simulink model "FlOWCITSS_3dof"  (R2019a)
settings: Solver=FixedStepAuto  StartTime=0.0  StopTime=15  FixedStep=0.00001  MaxStep=0.0001  RelTol=1e-5
values from neighbouring files (symbols this model uses):
  a11Inf = addedMassInf(1,4)    [FlOWCITSS.m]
  a13Inf = addedMassInf(2,4)    [FlOWCITSS.m]
  a15Inf = addedMassInf(3,4)    [FlOWCITSS.m]
  a31Inf = addedMassInf(4,4)    [FlOWCITSS.m]
  a33Inf = addedMassInf(5,4)    [FlOWCITSS.m]
  a35Inf = addedMassInf(6,4)    [FlOWCITSS.m]
  a51Inf = addedMassInf(7,4)    [FlOWCITSS.m]
  a53Inf = addedMassInf(8,4)    [FlOWCITSS.m]
  a55Inf = addedMassInf(9,4)    [FlOWCITSS.m]
  AH1 = full(SER.A)    [FlOWCITSS.m]
  AH3 = full(SER.A)    [FlOWCITSS.m]
  AH5 = full(SER.A)    [FlOWCITSS.m]
  AK11 = full(SER.A)    [FlOWCITSS.m]
  AK13 = full(SER.A)    [FlOWCITSS.m]
  AK15 = full(SER.A)    [FlOWCITSS.m]
  AK31 = full(SER.A)    [FlOWCITSS.m]
  AK33 = full(SER.A)    [FlOWCITSS.m]
  AK35 = full(SER.A)    [FlOWCITSS.m]
  AK51 = full(SER.A)    [FlOWCITSS.m]
  AK53 = full(SER.A)    [FlOWCITSS.m]
  AK55 = full(SER.A)    [FlOWCITSS.m]
  AY = full(SER.A)    [FlOWCITSS.m]
  BH1 = SER.B    [FlOWCITSS.m]
  BH3 = SER.B    [FlOWCITSS.m]
  BH5 = SER.B    [FlOWCITSS.m]
  BK11 = SER.B    [FlOWCITSS.m]
  BK13 = SER.B    [FlOWCITSS.m]
  BK15 = SER.B    [FlOWCITSS.m]
  BK31 = SER.B    [FlOWCITSS.m]
  BK33 = SER.B    [FlOWCITSS.m]
  BK35 = SER.B    [FlOWCITSS.m]
  BK51 = SER.B    [FlOWCITSS.m]
  BK53 = SER.B    [FlOWCITSS.m]
  BK55 = SER.B    [FlOWCITSS.m]
  BY = SER.B    [FlOWCITSS.m]
  C1inf = cInf(1,2)    [FlOWCITSS.m]
  C3inf = cInf(1,3)    [FlOWCITSS.m]
  C5inf = cInf(1,4)    [FlOWCITSS.m]
  CH1 = SER.C    [FlOWCITSS.m]
  CH3 = SER.C    [FlOWCITSS.m]
  CH5 = SER.C    [FlOWCITSS.m]
  CK11 = SER.C    [FlOWCITSS.m]
  CK13 = SER.C    [FlOWCITSS.m]
  CK15 = SER.C    [FlOWCITSS.m]
  CK31 = SER.C    [FlOWCITSS.m]
  CK33 = SER.C    [FlOWCITSS.m]
  CK35 = SER.C    [FlOWCITSS.m]
  CK51 = SER.C    [FlOWCITSS.m]
  CK53 = SER.C    [FlOWCITSS.m]
  CK55 = SER.C    [FlOWCITSS.m]
  CY = SER.C    [FlOWCITSS.m]
  DH1 = SER.D    [FlOWCITSS.m]
  DH3 = SER.D    [FlOWCITSS.m]
  DH5 = SER.D    [FlOWCITSS.m]
  DK11 = SER.D    [FlOWCITSS.m]
  DK13 = SER.D    [FlOWCITSS.m]
  DK15 = SER.D    [FlOWCITSS.m]
  DK31 = SER.D    [FlOWCITSS.m]
  DK33 = SER.D    [FlOWCITSS.m]
  DK35 = SER.D    [FlOWCITSS.m]
  DK51 = SER.D    [FlOWCITSS.m]
  DK53 = SER.D    [FlOWCITSS.m]
  DK55 = SER.D    [FlOWCITSS.m]
  DY = SER.D    [FlOWCITSS.m]
  gamma = 1.4    [FlOWCITSS_inputs.m]
  I5 = 1/(4.1625*10^8)    (= 2.4024024024e-09)    [FlOWCITSS_inputs.m]
  Mm = 1/(2.0270*10^6)    (= 4.93339911199e-07)    [FlOWCITSS_inputs.m]
  p0 = 101325    [FlOWCITSS_inputs.m]
  r1 = internalArea*0    (= 0)    [FlOWCITSS_inputs.m]
  r3 = internalArea*1    (= 472.5)    [FlOWCITSS_inputs.m]
  r5 = -internalArea*(5)    (= -2362.5)    [FlOWCITSS_inputs.m]
  Re = 10    [FlOWCITSS_inputs.m]
  Red1 = 91000    [FlOWCITSS_inputs.m]
  Red3 = 619000    [FlOWCITSS_inputs.m]
  Red5 = 190000000    [FlOWCITSS_inputs.m]
  Rq1 = rho*A1*Cd1    (= 1181250)    [FlOWCITSS_inputs.m]
  Rq3 = rho*A3*Cd3    (= 4725000)    [FlOWCITSS_inputs.m]
  Rq5 = 0    [FlOWCITSS_inputs.m]
  Ru = 20    [FlOWCITSS_inputs.m]
  SbS1 = +488000    (= 488000)    [FlOWCITSS_inputs.m]
  SbS3 = hydrostatics.data(15,3)*(rho*g*(ULEN^2))+11100    [FlOWCITSS_inputs.m]
  SbS35 = hydrostatics.data(17,3)*(rho*g*(ULEN^3))    [FlOWCITSS_inputs.m]
  SbS5 = hydrostatics.data(29,3)*(rho*g*(ULEN^4))+9920000    [FlOWCITSS_inputs.m]
  SbS53 = hydrostatics.data(27,3)*(rho*g*(ULEN^3))    [FlOWCITSS_inputs.m]
  V0 = 27*17.5*10    (= 4725)    [FlOWCITSS_inputs.m]
libraries: simulink x13
settings Model: Creator=huffl  LastModifiedBy=huffl
settings SolverCC: ZeroCrossAlgorithm=Adaptive

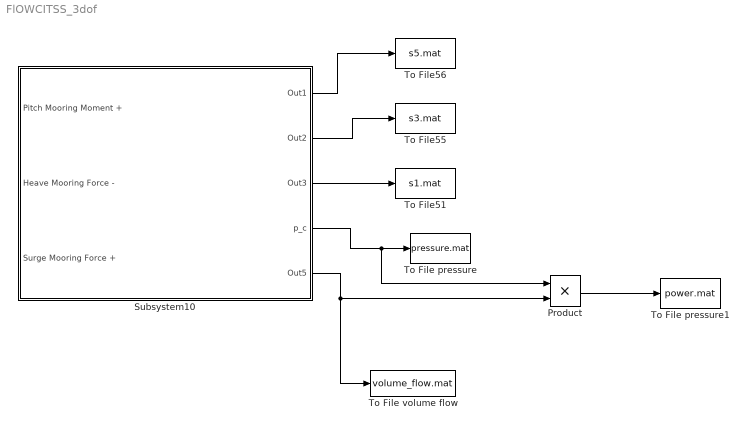
== system FlOWCITSS_3dof ==
  Product : Product
  Subsystem10 : Subsystem
  To File pressure : ToFile  Filename=pressure.mat  MatrixName=p_c  SaveFormat=Timeseries
  To File pressure1 : ToFile  Filename=power.mat  MatrixName=pneumaticPower  SaveFormat=Timeseries
  To File volume flow : ToFile  Filename=volume_flow.mat  MatrixName=Q_turbine  SaveFormat=Timeseries
  To File51 : ToFile  Filename=s1.mat  MatrixName=s1  SaveFormat=Timeseries
  To File55 : ToFile  Filename=s3.mat  MatrixName=s3  SaveFormat=Timeseries
  To File56 : ToFile  Filename=s5.mat  MatrixName=s5  SaveFormat=Timeseries
  wires:
  Subsystem10/1(Out1) -> To File56/1
  Subsystem10/2(Out2) -> To File55/1
  Subsystem10/3(Out3) -> To File51/1
  Subsystem10/4(p_c) -> Product/1, To File pressure/1
  Subsystem10/5(Out5) -> To File volume flow/1, Product/2
  Product/1 -> To File pressure1/1

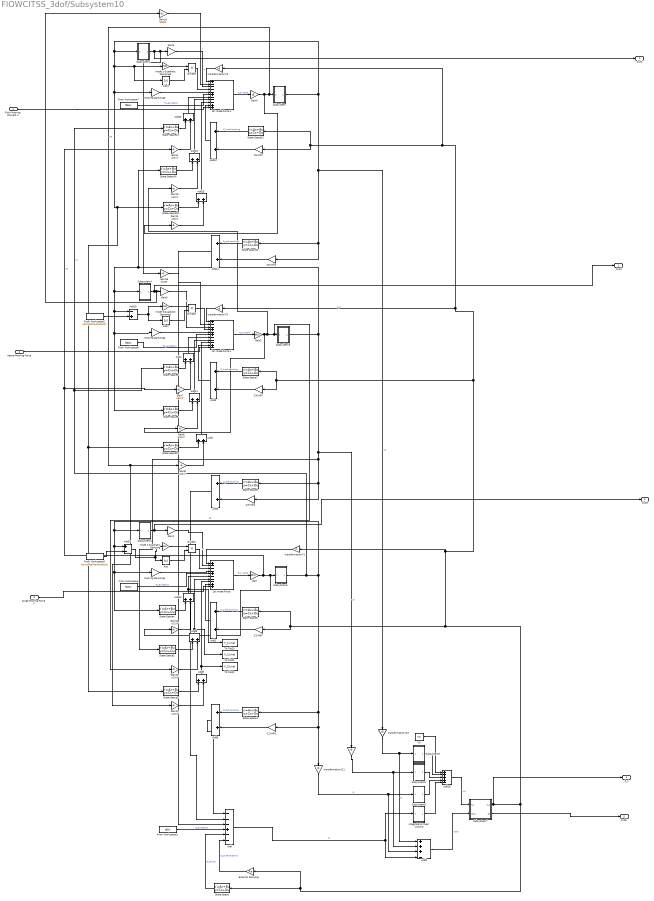
== system FlOWCITSS_3dof/Subsystem10 ==
  Pitch Mooring Moment + : Inport
  Heave Mooring Force - : Inport  Port=2
  "Surge Mooring Force + " : Inport  Port=3
  " " : Gain  Gain=r3
  "1st mode Force " : Sum  Inputs=+---+---++
  1st mode Force 1 : Sum  Inputs=+--+-+---+-
  1st mode Force 2 : Sum  Inputs=+----+---++
  Abs : Abs
  Abs2 : Abs
  Abs3 : Abs
  Add : Sum  Inputs=---+--
  Add{1,3..16} (15 alike) : Sum
  Add18 : Sum  Inputs=++++-
  Add19 : Sum  Inputs=-+
  Add2 : Sum  Inputs=+++-
  Add20 : Sum  Inputs=+-
  C1(inf)F : Gain  Gain=C1inf
  C1(inf)Q : Gain  Gain=C1inf
  C3(inf)F : Gain  Gain=C3inf
  C3(inf)Q : Gain  Gain=C3inf
  C5(inf)F : Gain  Gain=C5inf
  C5(inf)Q : Gain  Gain=C5inf
  Divide1 : Product  Inputs=**
  Divide2 : Product  Inputs=**
  Divide3 : Product  Inputs=**
  External Damping : Gain  Gain=Re
  From Workspace : FromWorkspace  VariableName=f1Exc  SampleTime=0
  From Workspace1 : FromWorkspace  VariableName=qExc  SampleTime=0
  From Workspace2 : FromWorkspace  VariableName=verticalWaveVelocity  SampleTime=0
  From Workspace3 : FromWorkspace  VariableName=horizontalWaveVelocity  SampleTime=0
  From Workspace6 : FromWorkspace  VariableName=f3Exc  SampleTime=0
  From Workspace7 : FromWorkspace  VariableName=f5Exc  SampleTime=0
  Gain : Gain  Gain=Mm
  Gain1 : Gain  Gain=SbS1
  Gain10 : Gain  Gain=a53Inf
  Gain11 : Gain  Gain=a55Inf
  Gain12 : Gain  Gain=a15Inf
  Gain13 : Gain  Gain=a13Inf
  Gain14 : Gain  Gain=a11Inf
  Gain15 : Gain  Gain=SbS35
  Gain16 : Gain  Gain=SbS53
  Gain2 : Gain  Gain=Mm
  Gain3 : Gain  Gain=SbS3
  Gain4 : Gain  Gain=I5
  Gain5 : Gain  Gain=SbS5
  Gain6 : Gain  Gain=a33Inf
  Gain7 : Gain  Gain=a31Inf
  Gain8 : Gain  Gain=a35Inf
  Gain9 : Gain  Gain=a51Inf
  "Integrate to creat Volume " : Subsystem
  Mooring Damping1 : Gain  Gain=Red1
  Mooring Damping2 : Gain  Gain=Red3
  Mooring Damping3 : Gain  Gain=Red5
  State-Space : StateSpace  A=AY  B=BY  C=CY  D=DY  InitialCondition=0
  State-Space1 : StateSpace  A=AH1  B=BH1  C=CH1  D=DH1  InitialCondition=0
  State-Space10 : StateSpace  A=AK35  B=BK35  C=CK35  D=DK35  InitialCondition=0
  State-Space11 : StateSpace  A=AH5  B=BH5  C=CH5  D=DH5  InitialCondition=0
  State-Space12 : StateSpace  A=AH5  B=BH5  C=CH5  D=DH5  InitialCondition=0
  State-Space13 : StateSpace  A=AK51  B=BK51  C=CK51  D=DK51  InitialCondition=0
  State-Space14 : StateSpace  A=AK53  B=BK53  C=CK53  D=DK53  InitialCondition=0
  State-Space15 : StateSpace  A=AK55  B=BK55  C=CK55  D=DK55  InitialCondition=0
  State-Space2 : StateSpace  A=AK15  B=BK15  C=CK15  D=DK15  InitialCondition=0
  State-Space3 : StateSpace  A=AK13  B=BK13  C=CK13  D=DK13  InitialCondition=0
  State-Space4 : StateSpace  A=AK11  B=BK11  C=CK11  D=DK11  InitialCondition=0
  State-Space5 : StateSpace  A=AH1  B=BH1  C=CH1  D=DH1  InitialCondition=0
  State-Space6 : StateSpace  A=AH3  B=BH3  C=CH3  D=DH3  InitialCondition=0
  State-Space7 : StateSpace  A=AH3  B=BH3  C=CH3  D=DH3  InitialCondition=0
  State-Space8 : StateSpace  A=AK31  B=BK31  C=CK31  D=DK31  InitialCondition=0
  State-Space9 : StateSpace  A=AK33  B=BK33  C=CK33  D=DK33  InitialCondition=0
  Subsystem : Subsystem
  Subsystem1 : Subsystem
  Subsystem2 : Subsystem
  Subsystem3 : Subsystem
  Subsystem4 : Subsystem
  Subsystem5 : Subsystem
  Subsystem6 : Subsystem
  Subsystem7 : Subsystem
  Subsystem8 : Subsystem
  Subsystem9 : Subsystem
  To File20 : ToFile  Filename=F_11.mat  MatrixName=F_11  SaveFormat=Timeseries
  To File21 : ToFile  Filename=F_13.mat  MatrixName=F_13  SaveFormat=Timeseries
  To File22 : ToFile  Filename=F_15.mat  MatrixName=F_15  SaveFormat=Timeseries
  V0 : Constant  Value=V0  VectorParams1D=off
  mode 1 Quadratic Damping : Gain  Gain=Rq1
  mode 1 Quadratic Damping2 : Gain  Gain=Rq5
  mode 3 Quadratic Damping1 : Gain  Gain=Rq3
  transformation F1 : Gain  Gain=r1
  transformation F2 : Gain  Gain=r3
  transformation F3 : Gain  Gain=r5
  transformation Q1 : Gain  Gain=r1
  transformation Q3 : Gain  Gain=r5
  Out1 : Outport
  Out2 : Outport  Port=2
  Out3 : Outport  Port=3
  p_c : Outport  Port=4
  Out5 : Outport  Port=5
  wires:
  Gain1/1 -> "1st mode Force "/2  "s"
  Add4/1 -> 1st mode Force 1/7
  Add2/1 -> Subsystem7/2(Vdot)  "Vdot"
  Add12/1 -> 1st mode Force 2/10
  Abs2/1 -> Divide2/2
  Add5/1 -> Add/2
  Add20/1 -> Abs/1, mode 1 Quadratic Damping/1
  1st mode Force 1/1 -> Gain2/1  "F_3 inertia"
  transformation Q3/1 -> Subsystem6/1(In1), Add2/1  "Q"
  Gain4/1 -> Gain11/1, Subsystem/1(In1), Gain12/1, Gain8/1  "a5"
  Divide3/1 -> 1st mode Force 2/4
  Add19/1 -> Abs2/1, mode 3 Quadratic Damping1/1
  C1(inf)Q/1 -> Add6/2
  Add9/1 -> To File21/1, "1st mode Force "/7
  Mooring Damping1/1 -> "1st mode Force "/4
  Subsystem5/1(Out1) -> State-Space13/1, State-Space8/1, transformation Q1/1, C1(inf)Q/1, State-Space1/1, Subsystem1/1(In1), Add20/1, State-Space4/1, Mooring Damping1/1  "u1"
  Add8/1 -> To File22/1, "1st mode Force "/8
  Gain2/1 -> Gain6/1, Gain10/1, Subsystem3/1(In1), Gain13/1  "a3"
  Add16/1 -> 1st mode Force 2/8
  C5(inf)Q/1 -> Add14/2
  Add18/1 -> Subsystem7/1(V_c)  "V_c"
  State-Space7/1 -> Add3/1  "F_1 rad.coupling"
  State-Space14/1 -> Add16/1
  Divide2/1 -> 1st mode Force 1/4
  Subsystem1/1(Out1) -> Out3/1, Gain1/1
  V0/1 -> Add18/1
  State-Space8/1 -> Add4/1
  transformation Q1/1 -> Add2/3, Subsystem8/1(In1)  "Q"
  State-Space6/1 -> Add5/1  "Q_rad.coupling"
  Add/1 -> Add2/4, "Integrate to creat Volume "/1(In1)  "Q"
  Gain15/1 -> 1st mode Force 1/2
  Gain7/1 -> Add4/2
  Add7/1 -> 1st mode Force 1/9
  State-Space5/1 -> Add1/1  "F_1 rad.coupling"
  Subsystem3/1(Out1) -> " "/1, State-Space3/1, State-Space6/1, C3(inf)Q/1, State-Space14/1, Subsystem4/1(In1), Add19/1, State-Space9/1, Mooring Damping2/1  "u3"
  From Workspace1/1 -> Add/4  "Q_excitation"
  Gain12/1 -> Add8/2
  State-Space10/1 -> Add7/1
  Add3/1 -> 1st mode Force 1/10
  "1st mode Force "/1 -> Gain/1  "F_1 inertia"
  Gain6/1 -> Add11/2
  Abs3/1 -> Divide3/2
  Subsystem7/1(p_c) -> p_c/1, External Damping/1, State-Space/1, transformation F3/1, State-Space12/1, C5(inf)F/1, transformation F2/1, State-Space7/1, C3(inf)F/1, transformation F1/1, State-Space5/1, C1(inf)F/1  "p_c"
  Subsystem/1(Out1) -> Subsystem2/1(In1), Mooring Damping3/1, State-Space15/1, State-Space2/1, State-Space10/1, Abs3/1, mode 1 Quadratic Damping2/1, transformation Q3/1, State-Space11/1, C5(inf)Q/1  "u5"
  State-Space2/1 -> Add8/1
  Abs/1 -> Divide1/2
  State-Space3/1 -> Add9/1
  Gain13/1 -> Add9/2
  State-Space1/1 -> Add6/1  "Q_rad.coupling"
  Add10/1 -> To File20/1, "1st mode Force "/6
  mode 3 Quadratic Damping1/1 -> Divide2/1
  External Damping/1 -> Add/6  "Q_externaldamp"
  State-Space12/1 -> Add12/1  "F_1 rad.coupling"
  State-Space13/1 -> Add13/1
  transformation F2/1 -> 1st mode Force 1/1
  Gain/1 -> Subsystem5/1(In1), Gain14/1, Gain9/1, Gain7/1  "a1"
  State-Space/1 -> Add/5  "Q_rad.ad"
  State-Space11/1 -> Add14/1  "Q_rad.coupling"
  transformation F1/1 -> "1st mode Force "/1
  State-Space15/1 -> Add15/1
  State-Space4/1 -> Add10/1
  From Workspace/1 -> "1st mode Force "/5  "F1_excitation"
  State-Space9/1 -> Add11/1
  Add11/1 -> 1st mode Force 1/8
  Gain10/1 -> Add16/2
  mode 1 Quadratic Damping2/1 -> Divide3/1
  C3(inf)F/1 -> Add3/2
  Gain9/1 -> Add13/2
  C3(inf)Q/1 -> Add5/2
  From Workspace6/1 -> 1st mode Force 1/6  "F1_excitation"
  Gain14/1 -> Add10/2
  transformation F3/1 -> 1st mode Force 2/1
  Mooring Damping3/1 -> 1st mode Force 2/5
  Gain11/1 -> Add15/2
  C5(inf)F/1 -> Add12/2
  Gain5/1 -> 1st mode Force 2/3  "s"
  From Workspace7/1 -> 1st mode Force 2/6  "F1_excitation"
  Add1/1 -> "1st mode Force "/9
  Add13/1 -> 1st mode Force 2/7
  Add15/1 -> 1st mode Force 2/9
  Add14/1 -> Add/3
  1st mode Force 2/1 -> Gain4/1  "F_5 inertia"
  Subsystem6/1(Out1) -> Add18/2
  Subsystem8/1(Out1) -> Add18/4
  Subsystem9/1(Out1) -> Add18/3
  Add6/1 -> Add/1
  "Integrate to creat Volume "/1(Out1) -> Add18/5
  Subsystem4/1(Out1) -> Out2/1, Gain16/1, Gain3/1
  Divide1/1 -> "1st mode Force "/3
  Gain8/1 -> Add7/2
  Mooring Damping2/1 -> 1st mode Force 1/5
  " "/1 -> Subsystem9/1(In1), Add2/2
  mode 1 Quadratic Damping/1 -> Divide1/1
  Gain16/1 -> 1st mode Force 2/2  "s"
  Subsystem2/1(Out1) -> Out1/1, Gain15/1, Gain5/1
  From Workspace3/1 -> Add20/2
  From Workspace2/1 -> Add19/2
  C1(inf)F/1 -> Add1/2
  Gain3/1 -> 1st mode Force 1/3  "s"
  Heave Mooring Force -/1 -> 1st mode Force 1/11
  Pitch Mooring Moment +/1 -> 1st mode Force 2/11
  "Surge Mooring Force + "/1 -> "1st mode Force "/10
  Subsystem7/2("Qt ") -> Out5/1

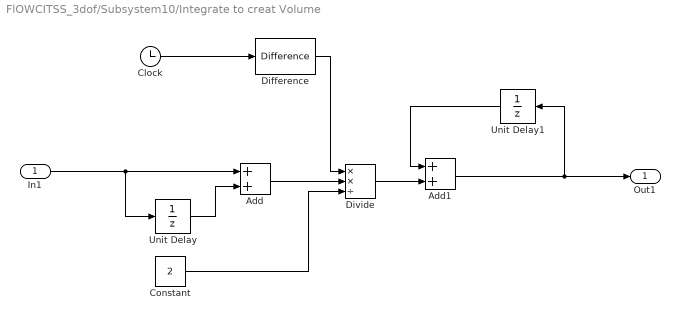
== system FlOWCITSS_3dof/Subsystem10/Integrate to creat Volume  ==
  In1 : Inport
  Add : Sum
  Add1 : Sum
  Clock : Clock
  Constant : Constant  Value=2
  Difference : simulink/Discrete/Difference  ICPrevInput=0.0  OutMin=[]  OutMax=[]  OutDataType=fixdt(1, 16)  OutScaling=2^-10  DoSatur=off
  Divide : Product  Inputs=**/
  Unit Delay : UnitDelay  SampleTime=-1  HasFrameUpgradeWarning=on
  Unit Delay1 : UnitDelay  SampleTime=-1  HasFrameUpgradeWarning=on
  Out1 : Outport
  wires:
  Add1/1 -> Out1/1, Unit Delay1/1
  Add/1 -> Divide/2
  Unit Delay1/1 -> Add1/1
  Constant/1 -> Divide/3
  Divide/1 -> Add1/2
  In1/1 -> Unit Delay/1, Add/1
  Difference/1 -> Divide/1
  Unit Delay/1 -> Add/2
  Clock/1 -> Difference/1

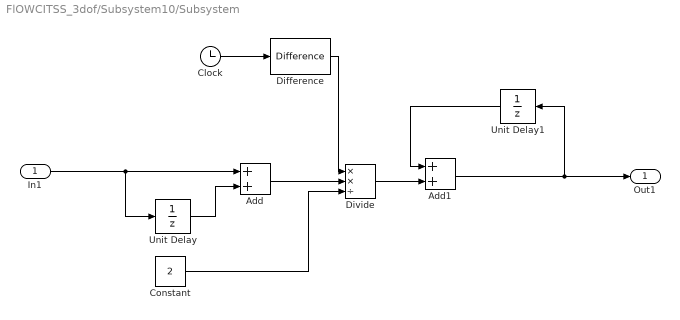
== system FlOWCITSS_3dof/Subsystem10/Subsystem ==
  In1 : Inport
  Add : Sum
  Add1 : Sum
  Clock : Clock
  Constant : Constant  Value=2
  Difference : simulink/Discrete/Difference  ICPrevInput=0.0  OutMin=[]  OutMax=[]  OutDataType=fixdt(1, 16)  OutScaling=2^-10  DoSatur=off
  Divide : Product  Inputs=**/
  Unit Delay : UnitDelay  SampleTime=-1  HasFrameUpgradeWarning=on
  Unit Delay1 : UnitDelay  SampleTime=-1  HasFrameUpgradeWarning=on
  Out1 : Outport
  wires:
  Add1/1 -> Out1/1, Unit Delay1/1
  Add/1 -> Divide/2
  Unit Delay1/1 -> Add1/1
  Clock/1 -> Difference/1
  Constant/1 -> Divide/3
  Divide/1 -> Add1/2
  In1/1 -> Unit Delay/1, Add/1
  Difference/1 -> Divide/1
  Unit Delay/1 -> Add/2

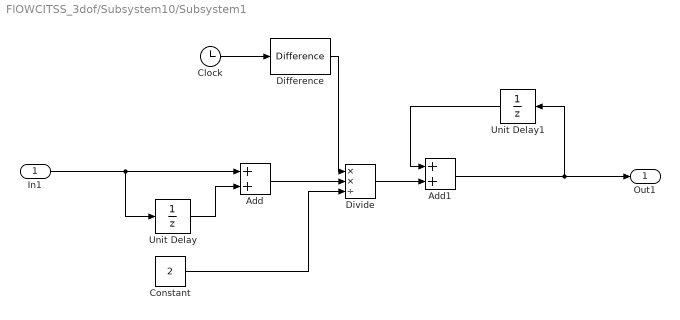
== system FlOWCITSS_3dof/Subsystem10/Subsystem1 ==
  In1 : Inport
  Add : Sum
  Add1 : Sum
  Clock : Clock
  Constant : Constant  Value=2
  Difference : simulink/Discrete/Difference  ICPrevInput=0.0  OutMin=[]  OutMax=[]  OutDataType=fixdt(1, 16)  OutScaling=2^-10  DoSatur=off
  Divide : Product  Inputs=**/
  Unit Delay : UnitDelay  SampleTime=-1  HasFrameUpgradeWarning=on
  Unit Delay1 : UnitDelay  SampleTime=-1  HasFrameUpgradeWarning=on
  Out1 : Outport
  wires:
  Add1/1 -> Out1/1, Unit Delay1/1
  Add/1 -> Divide/2
  Unit Delay1/1 -> Add1/1
  Clock/1 -> Difference/1
  Constant/1 -> Divide/3
  Divide/1 -> Add1/2
  In1/1 -> Unit Delay/1, Add/1
  Difference/1 -> Divide/1
  Unit Delay/1 -> Add/2

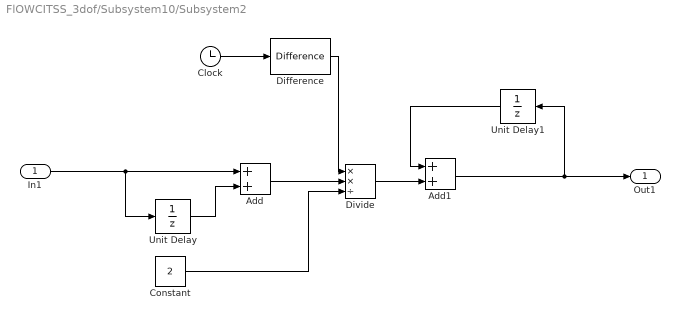
== system FlOWCITSS_3dof/Subsystem10/Subsystem2 ==
  In1 : Inport
  Add : Sum
  Add1 : Sum
  Clock : Clock
  Constant : Constant  Value=2
  Difference : simulink/Discrete/Difference  ICPrevInput=0.0  OutMin=[]  OutMax=[]  OutDataType=fixdt(1, 16)  OutScaling=2^-10  DoSatur=off
  Divide : Product  Inputs=**/
  Unit Delay : UnitDelay  SampleTime=-1  HasFrameUpgradeWarning=on
  Unit Delay1 : UnitDelay  SampleTime=-1  HasFrameUpgradeWarning=on
  Out1 : Outport
  wires:
  Add1/1 -> Out1/1, Unit Delay1/1
  Add/1 -> Divide/2
  Unit Delay1/1 -> Add1/1
  Clock/1 -> Difference/1
  Constant/1 -> Divide/3
  Divide/1 -> Add1/2
  In1/1 -> Unit Delay/1, Add/1
  Difference/1 -> Divide/1
  Unit Delay/1 -> Add/2

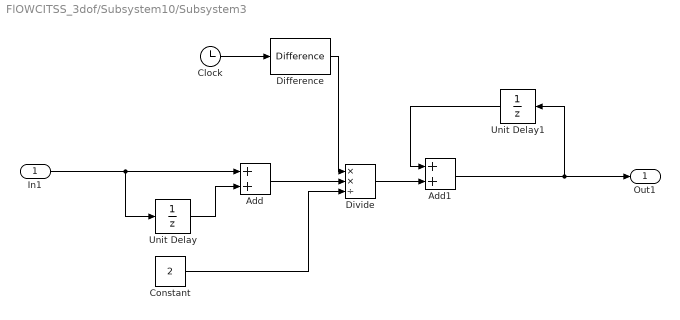
== system FlOWCITSS_3dof/Subsystem10/Subsystem3 ==
  In1 : Inport
  Add : Sum
  Add1 : Sum
  Clock : Clock
  Constant : Constant  Value=2
  Difference : simulink/Discrete/Difference  ICPrevInput=0.0  OutMin=[]  OutMax=[]  OutDataType=fixdt(1, 16)  OutScaling=2^-10  DoSatur=off
  Divide : Product  Inputs=**/
  Unit Delay : UnitDelay  SampleTime=-1  HasFrameUpgradeWarning=on
  Unit Delay1 : UnitDelay  SampleTime=-1  HasFrameUpgradeWarning=on
  Out1 : Outport
  wires:
  Add1/1 -> Out1/1, Unit Delay1/1
  Add/1 -> Divide/2
  Unit Delay1/1 -> Add1/1
  Clock/1 -> Difference/1
  Constant/1 -> Divide/3
  Divide/1 -> Add1/2
  In1/1 -> Unit Delay/1, Add/1
  Difference/1 -> Divide/1
  Unit Delay/1 -> Add/2

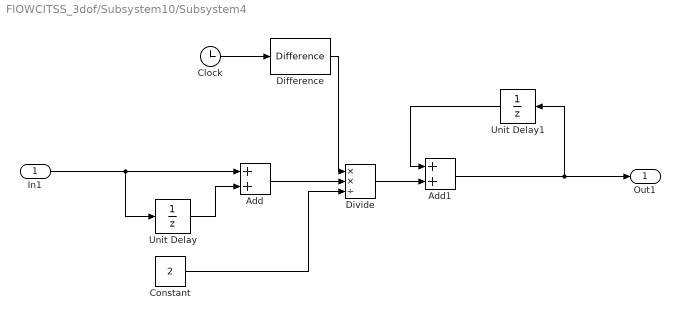
== system FlOWCITSS_3dof/Subsystem10/Subsystem4 ==
  In1 : Inport
  Add : Sum
  Add1 : Sum
  Clock : Clock
  Constant : Constant  Value=2
  Difference : simulink/Discrete/Difference  ICPrevInput=0.0  OutMin=[]  OutMax=[]  OutDataType=fixdt(1, 16)  OutScaling=2^-10  DoSatur=off
  Divide : Product  Inputs=**/
  Unit Delay : UnitDelay  SampleTime=-1  HasFrameUpgradeWarning=on
  Unit Delay1 : UnitDelay  SampleTime=-1  HasFrameUpgradeWarning=on
  Out1 : Outport
  wires:
  Add1/1 -> Out1/1, Unit Delay1/1
  Add/1 -> Divide/2
  Unit Delay1/1 -> Add1/1
  Clock/1 -> Difference/1
  Constant/1 -> Divide/3
  Divide/1 -> Add1/2
  In1/1 -> Unit Delay/1, Add/1
  Difference/1 -> Divide/1
  Unit Delay/1 -> Add/2

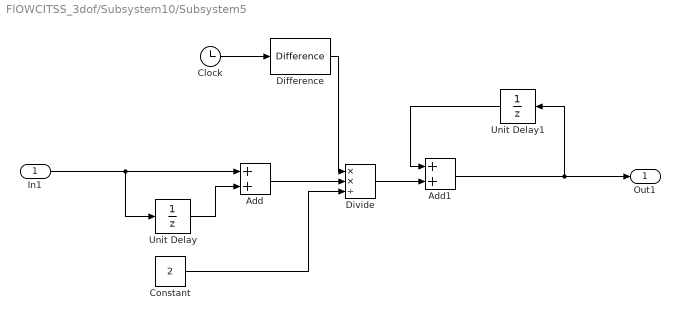
== system FlOWCITSS_3dof/Subsystem10/Subsystem5 ==
  In1 : Inport
  Add : Sum
  Add1 : Sum
  Clock : Clock
  Constant : Constant  Value=2
  Difference : simulink/Discrete/Difference  ICPrevInput=0.0  OutMin=[]  OutMax=[]  OutDataType=fixdt(1, 16)  OutScaling=2^-10  DoSatur=off
  Divide : Product  Inputs=**/
  Unit Delay : UnitDelay  SampleTime=-1  HasFrameUpgradeWarning=on
  Unit Delay1 : UnitDelay  SampleTime=-1  HasFrameUpgradeWarning=on
  Out1 : Outport
  wires:
  Add1/1 -> Out1/1, Unit Delay1/1
  Add/1 -> Divide/2
  Unit Delay1/1 -> Add1/1
  Clock/1 -> Difference/1
  Constant/1 -> Divide/3
  Divide/1 -> Add1/2
  In1/1 -> Unit Delay/1, Add/1
  Difference/1 -> Divide/1
  Unit Delay/1 -> Add/2

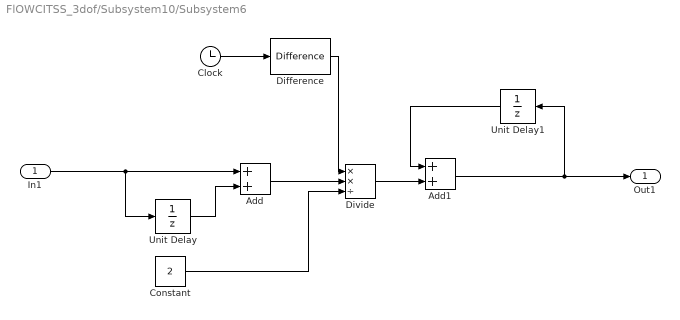
== system FlOWCITSS_3dof/Subsystem10/Subsystem6 ==
  In1 : Inport
  Add : Sum
  Add1 : Sum
  Clock : Clock
  Constant : Constant  Value=2
  Difference : simulink/Discrete/Difference  ICPrevInput=0.0  OutMin=[]  OutMax=[]  OutDataType=fixdt(1, 16)  OutScaling=2^-10  DoSatur=off
  Divide : Product  Inputs=**/
  Unit Delay : UnitDelay  SampleTime=-1  HasFrameUpgradeWarning=on
  Unit Delay1 : UnitDelay  SampleTime=-1  HasFrameUpgradeWarning=on
  Out1 : Outport
  wires:
  Add1/1 -> Out1/1, Unit Delay1/1
  Add/1 -> Divide/2
  Unit Delay1/1 -> Add1/1
  Clock/1 -> Difference/1
  Constant/1 -> Divide/3
  Divide/1 -> Add1/2
  In1/1 -> Unit Delay/1, Add/1
  Difference/1 -> Divide/1
  Unit Delay/1 -> Add/2

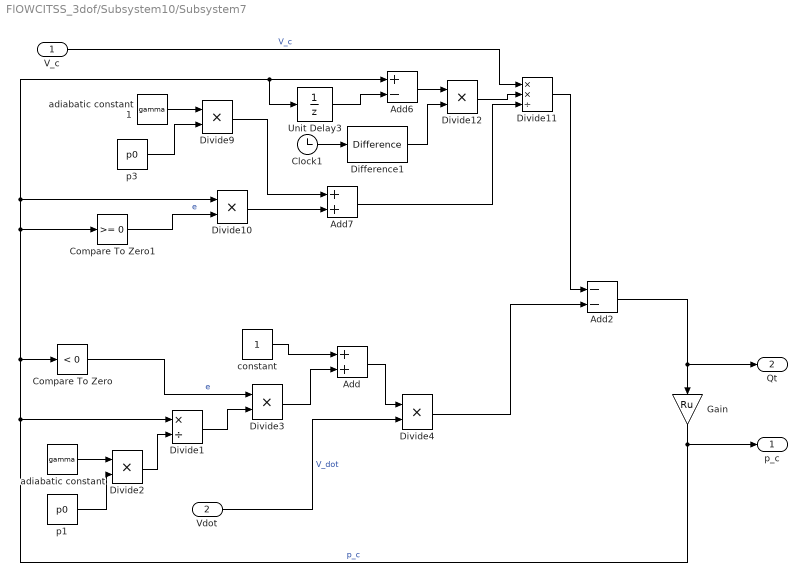
== system FlOWCITSS_3dof/Subsystem10/Subsystem7 ==
  V_c : Inport
  Vdot : Inport  Port=2
  Add : Sum
  Add2 : Sum  Inputs=--
  Add6 : Sum  Inputs=+-
  Add7 : Sum
  Clock1 : Clock
  Compare To Zero : simulink/Logic and Bit Operations/Compare To Zero  relop=<  OutDataTypeStr=boolean
  Compare To Zero1 : simulink/Logic and Bit Operations/Compare To Zero  relop=>=  OutDataTypeStr=boolean
  Difference1 : simulink/Discrete/Difference  ICPrevInput=0.0  OutMin=[]  OutMax=[]  OutDataType=fixdt(1, 16)  OutScaling=2^-10  DoSatur=off
  Divide1 : Product  Inputs=*/
  Divide{2..4,9..10,12} (6 alike) : Product  Inputs=**
  Divide11 : Product  Inputs=**/
  Gain : Gain  Gain=Ru
  Unit Delay3 : UnitDelay  SampleTime=-1  HasFrameUpgradeWarning=on
  "adiabatic constant " : Constant  Value=gamma  VectorParams1D=off
  adiabatic constant 1 : Constant  Value=gamma  VectorParams1D=off
  constant : Constant
  p1 : Constant  Value=p0
  p3 : Constant  Value=p0
  p_c : Outport
  "Qt " : Outport  Port=2
  wires:
  Compare To Zero/1 -> Divide3/1  "e"
  Gain/1 -> Compare To Zero/1, Compare To Zero1/1, Divide10/1, Unit Delay3/1, Add6/1, Divide1/1, p_c/1  "p_c"
  V_c/1 -> Divide11/1  "V_c"
  constant/1 -> Add/1
  Divide1/1 -> Divide3/2
  "adiabatic constant "/1 -> Divide2/1
  Divide2/1 -> Divide1/2
  p1/1 -> Divide2/2
  Vdot/1 -> Divide4/2  "V_dot"
  adiabatic constant 1/1 -> Divide9/1
  p3/1 -> Divide9/2
  Divide9/1 -> Add7/1
  Divide10/1 -> Add7/2
  Unit Delay3/1 -> Add6/2
  Add6/1 -> Divide12/1
  Clock1/1 -> Difference1/1
  Difference1/1 -> Divide12/2
  Divide12/1 -> Divide11/2
  Divide11/1 -> Add2/1
  Add2/1 -> Gain/1, "Qt "/1
  Add7/1 -> Divide11/3
  Divide3/1 -> Add/2
  Add/1 -> Divide4/1
  Compare To Zero1/1 -> Divide10/2  "e"
  Divide4/1 -> Add2/2

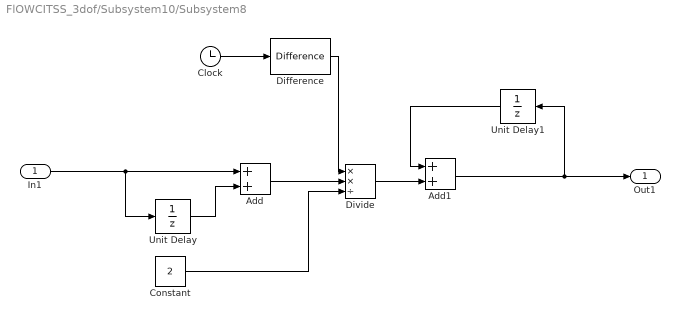
== system FlOWCITSS_3dof/Subsystem10/Subsystem8 ==
  In1 : Inport
  Add : Sum
  Add1 : Sum
  Clock : Clock
  Constant : Constant  Value=2
  Difference : simulink/Discrete/Difference  ICPrevInput=0.0  OutMin=[]  OutMax=[]  OutDataType=fixdt(1, 16)  OutScaling=2^-10  DoSatur=off
  Divide : Product  Inputs=**/
  Unit Delay : UnitDelay  SampleTime=-1  HasFrameUpgradeWarning=on
  Unit Delay1 : UnitDelay  SampleTime=-1  HasFrameUpgradeWarning=on
  Out1 : Outport
  wires:
  Add1/1 -> Out1/1, Unit Delay1/1
  Add/1 -> Divide/2
  Unit Delay1/1 -> Add1/1
  Clock/1 -> Difference/1
  Constant/1 -> Divide/3
  Divide/1 -> Add1/2
  In1/1 -> Unit Delay/1, Add/1
  Difference/1 -> Divide/1
  Unit Delay/1 -> Add/2

== system FlOWCITSS_3dof/Subsystem10/Subsystem9 ==
  In1 : Inport
  Add : Sum
  Add1 : Sum
  Clock : Clock
  Constant : Constant  Value=2
  Difference : simulink/Discrete/Difference  ICPrevInput=0.0  OutMin=[]  OutMax=[]  OutDataType=fixdt(1, 16)  OutScaling=2^-10  DoSatur=off
  Divide : Product  Inputs=**/
  Unit Delay : UnitDelay  SampleTime=-1  HasFrameUpgradeWarning=on
  Unit Delay1 : UnitDelay  SampleTime=-1  HasFrameUpgradeWarning=on
  Out1 : Outport
  wires:
  Add1/1 -> Out1/1, Unit Delay1/1
  Add/1 -> Divide/2
  Unit Delay1/1 -> Add1/1
  Clock/1 -> Difference/1
  Constant/1 -> Divide/3
  Divide/1 -> Add1/2
  In1/1 -> Unit Delay/1, Add/1
  Difference/1 -> Divide/1
  Unit Delay/1 -> Add/2
